simulink model "Allgemein"  (R2021a)
settings: Solver=ode45  StartTime=0.0  StopTime=inf  RelTol=1e-3  EnableMultiTasking=on
undefined symbols (not defined in the file): samples_per_frame, sampling_frequency, visa_obj
libraries: dspsigattribs x3, dspstat3 x3
settings Model: Creator=MT-LAB  LastModifiedBy=MT-LAB
settings SolverCC: AlgebraicLoopSolver=TrustRegion
settings DataIOCC: LimitDataPoints=on  SaveFormat=Array  ReturnWorkspaceOutputs=off
settings OptimizationCC: LifeSpan=inf
settings DebuggingCC: UnderspecifiedInitializationDetection=Classic  MergeDetectMultiDrivingBlocksExec=none  SolverPrmCheckMsg=warning  SFUnexpectedBacktrackingDiag=warning  SFNoUnconditionalDefaultTransitionDiag=warning  SFExecutionAtInitializationDiag=none  SFMachineParentedDataDiag=warning  ArithmeticOperatorsInVariantConditions=warning
settings HardwareCC: ProdBitPerPointer=32  ProdBitPerSizeT=32  ProdBitPerPtrDiffT=32  ProdLargestAtomicFloat=None  ProdIntDivRoundTo=Undefined  ProdEndianess=Unspecified  ProdWordSize=32  ProdHWDeviceType=32-bit Generic
settings ModelReferenceCC: PropagateSignalLabelsOutOfModel=off
settings SFSimCC: SimUseLocalCustomCode=off  CustomCodeUndefinedFunction=UseInterfaceOnly
settings RTWCC: RTWUseLocalCustomCode=off
settings CodeAppCC: StateflowObjectComments=on
settings GRTTargetCC: TargetLangStandard=C89/C90 (ANSI)
settings ConfigComp: CovMetricSettings=dw  CovSaveCumulativeToWorkspaceVar=on  CovSaveSingleToWorkspaceVar=on  CovExternalEMLEnable=off

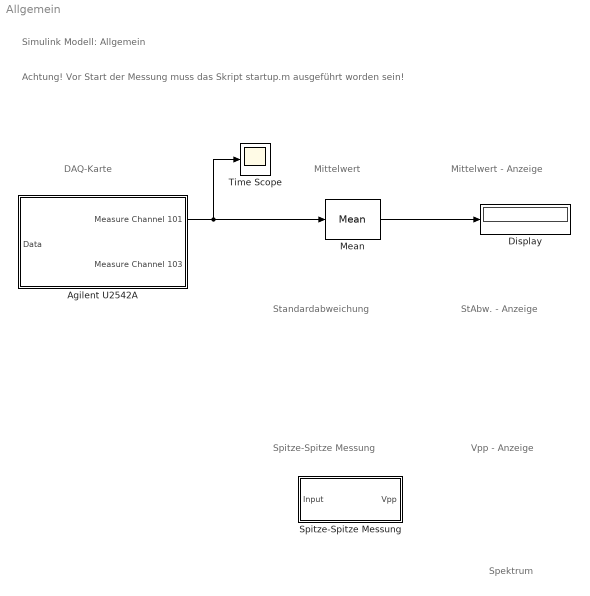
== system Allgemein ==
  note: Simulink Modell: Allgemein
  note: Mittelwert
  note: Mittelwert - Anzeige
  note: DAQ-Karte
  note: Standardabweichung
  note: Spitze-Spitze Messung
  note: StAbw. - Anzeige
  note: Vpp - Anzeige
  note: Achtung! Vor Start der Messung muss das Skript startup.m ausgeführt worden sein!
  note: Spektrum
  Agilent U2542A : Subsystem  mask(Agilent U2542A){visaaddr=USB0::0x0957::0x1718::TW53354503::0::INSTR, samplingtime=1/sampling_frequency, datapoints=samples_per_frame, input=AI101, output=AO201}
      mask prompts: visaaddr "Visa Address"; samplingtime "Sampling Time"; datapoints "Samples per Frame"; input "Input Channel"; output "Ouput Channel"
      mask help: Driver for the Agilent U2542A.
      mask TypeOptions input: AI101 | AI102 | AI103 | AI104
      mask TypeOptions output: AO201 | AO202
      mask Display:
      | port_label('output', 1, 'AI101')
      | port_label('output', 2, 'AI102')
      | port_label('input', 1, 'AO201')
      | fprintf('Agilent U2542A')
  Display : Display
  Mean : dspstat3/Mean  run=off  InputProcessing=Columns as channels (frame based)  reset_popup=None  directionMode=Each column  dimension=1  roiEnable=off  roiType=Rectangles  roiPortion=Entire ROI  roiOutput=Individual statistics for each ROI  roiFlag=off  roundingMode=Floor  overflowMode=off  outputDataTypeStr=Inherit: Same as accumulator  outputMin=[]  outputMax=[]  outputLastDataTypeStr=Inherit: Same as accumulator
  Spitze-Spitze Messung : Subsystem
  Time Scope : Scope
  wires:
  Agilent U2542A/1(Measure Channel 101) -> Mean/1, Time Scope/1
  Mean/1 -> Display/1

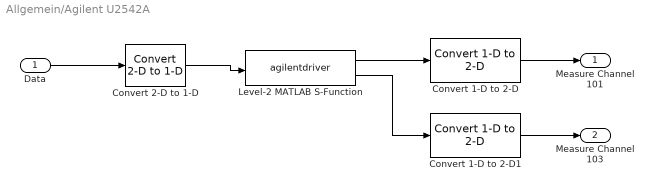
== system Allgemein/Agilent U2542A ==
  Data : Inport
  Convert 1-D to 2-D : dspsigattribs/Convert 1-D to 2-D  M=datapoints  N=1  frameBasedOut=on
      settings: SourceProductBaseCode=DS
  Convert 1-D to 2-D1 : dspsigattribs/Convert 1-D to 2-D  M=datapoints  N=1  frameBasedOut=on
      settings: SourceProductBaseCode=DS
  Convert 2-D to 1-D : dspsigattribs/Convert 2-D to 1-D
      settings: SourceProductBaseCode=DS
  Level-2 MATLAB S-Function : M-S-Function  FunctionName=agilentdriver  Parameters=samplingtime,datapoints,input,output,visaaddr,visa_obj
  Measure Channel 101 : Outport
  "Measure Channel 103 " : Outport  Port=2
  wires:
  Data/1 -> Convert 2-D to 1-D/1
  Convert 2-D to 1-D/1 -> Level-2 MATLAB S-Function/1
  Level-2 MATLAB S-Function/1 -> Convert 1-D to 2-D/1
  Convert 1-D to 2-D/1 -> Measure Channel 101/1
  Level-2 MATLAB S-Function/2 -> Convert 1-D to 2-D1/1
  Convert 1-D to 2-D1/1 -> "Measure Channel 103 "/1

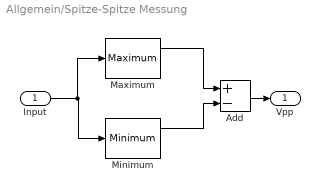
== system Allgemein/Spitze-Spitze Messung ==
  Input : Inport
  Add : Sum  Inputs=+-
  Maximum : dspstat3/Maximum  operation=maximum  fcn=Value and Index  indexBase=One  operateOver=Each column  Dimension=1  InputProcessing=Columns as channels (frame based)  reset=None  roiEnable=off  roiType=Rectangles  roiPortion=Entire ROI  roiOutput=Individual statistics for each ROI  roiFlag=off  roundingMode=Floor  overflowMode=off  accumDataTypeStr=Inherit: Same as product output  accumLastDataTypeStr=Inherit: Same as product output
  Minimum : dspstat3/Minimum  operation=minimum  fcn=Value and Index  indexBase=One  operateOver=Each column  Dimension=1  InputProcessing=Columns as channels (frame based)  reset=None  roiEnable=off  roiType=Rectangles  roiPortion=Entire ROI  roiOutput=Individual statistics for each ROI  roiFlag=off  roundingMode=Floor  overflowMode=off
      settings: SourceProductBaseCode=DS
  Vpp : Outport
  wires:
  Minimum/1 -> Add/2
  Maximum/1 -> Add/1
  Add/1 -> Vpp/1
  Input/1 -> Maximum/1, Minimum/1
